simulink model "nonlin_sim_task4"  (R2023a)
settings: Solver=VariableStepAuto  StartTime=0.0  StopTime=100  RelTol=1e-3
values from neighbouring files (symbols this model uses):
  La_La_La_La_c_at_x0_numeric = double(subs(La_La_La_La_c_at_x0, param_values, param_numeric))    [nonlin_lab_task4.m]    (also in nonlin_lab_task6.m)
  Lb_La_La_La_c_at_x0_numeric = double(subs(Lb_La_La_La_c_at_x0, param_values, param_numeric))    [nonlin_lab_task4.m]    (also in nonlin_lab_task6.m)
  x_init = [0 0 0 0]'    [nonlin_lab.m]    (also in nonlin_lab_task2.m = [0 0 theta_m_eq 0]'; nonlin_lab_task4.m = [0 0 theta_m_eq 0]'; nonlin_lab_task6.m = [0 0 theta_m_eq 0]')
undefined symbols (not defined in the file or in its folder): K_lin_feedback
settings Model: Creator=M4RTI  LastModifiedBy=M4RTI

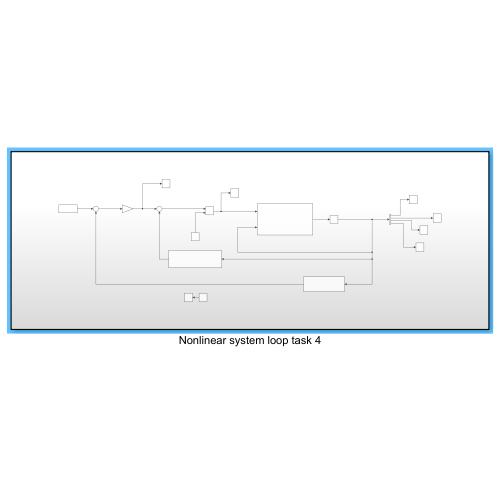
[thumbnail: Simulink's stored preview of the top-level diagram]
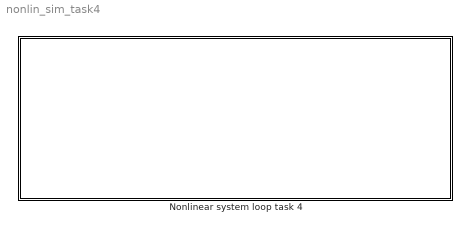
== system nonlin_sim_task4 ==
  Nonlinear system loop task 4 : Subsystem

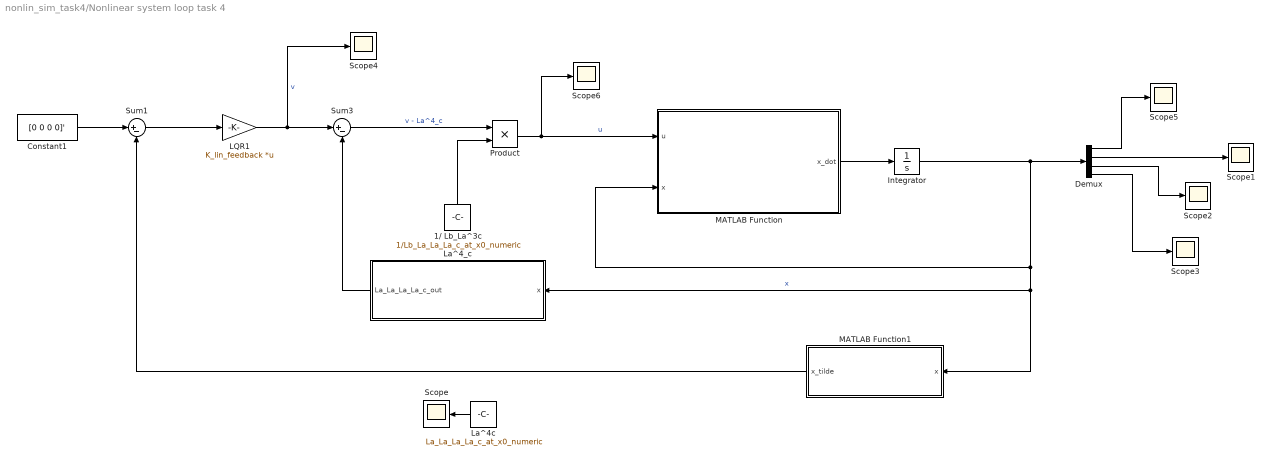
== system nonlin_sim_task4/Nonlinear system loop task 4 ==
  1/ Lb_La^3c : Constant  Value=1/Lb_La_La_La_c_at_x0_numeric
  Constant1 : Constant  Value=[0 0 0 0]'
  Demux : Demux
  Integrator : Integrator  InitialCondition=x_init
  LQR1 : Gain  Gain=K_lin_feedback  Multiplication=Matrix(K*u)
  La^4_c : MATLAB Function  TreatAsAtomicUnit=on
  La^4c : Constant  Value=La_La_La_La_c_at_x0_numeric
  MATLAB Function : MATLAB Function  TreatAsAtomicUnit=on
  MATLAB Function1 : MATLAB Function  TreatAsAtomicUnit=on
  Product : Product
  Scope{,1..6} (7 alike) : Scope
  Sum1 : Sum  Inputs=|+-
  Sum3 : Sum  Inputs=|+-
  wires:
  Demux/1 -> Scope5/1
  Demux/4 -> Scope3/1
  Integrator/1 -> Demux/1, MATLAB Function1/1(x), La^4_c/1(x), MATLAB Function/2(x)  "x"
  Demux/2 -> Scope1/1
  Demux/3 -> Scope2/1
  MATLAB Function/1(x_dot) -> Integrator/1
  Product/1 -> Scope6/1, MATLAB Function/1(u)  "u"
  LQR1/1 -> Scope4/1, Sum3/1  "v"
  Sum3/1 -> Product/1  "v - La^4_c"
  1/ Lb_La^3c/1 -> Product/2
  La^4c/1 -> Scope/1
  La^4_c/1(La_La_La_La_c_out) -> Sum3/2
  Sum1/1 -> LQR1/1
  Constant1/1 -> Sum1/1
  MATLAB Function1/1(x_tilde) -> Sum1/2

== matlab function nonlin_sim_task4/Nonlinear system loop task 4/MATLAB Function ==
  data: u input; x input; x_dot output
function x_dot = nonlin_system(u, x)
    m = 0.3;   % Mass of the load (kg)
    l = 0.3;   % Length to the center of mass of the load (m)
    g = 9.8;   % Acceleration due to gravity (m/s^2)
    J_l = 4e-4; % Moment of inertia of the load (Nms^2/rad)
    J_m = 4e-4; % Moment of inertia of the motor (Nms^2/rad)
    B_l = 0.0;  % Damping coefficient of the load (Nms/rad)
    B_m = 0.015; % Damping coefficient of the motor (Nms/rad)
    k = 0.8;    % Spring constant (Nm/rad)

    % Nonlinear dynamics
    theta_l = x(1);
    theta_l_dot = x(2);
    theta_m = x(3);
    theta_m_dot = x(4);

    x1_dot = theta_l_dot;
    x2_dot = -1/J_l * (B_l * theta_l_dot + k * (theta_l - theta_m) + m * g * l * cos(theta_l));
    x3_dot = theta_m_dot;
    x4_dot = 1/J_m * (u + k * (theta_l - theta_m) - B_m * theta_m_dot);

    % Output: the derivatives of the state variables
    x_dot = [x1_dot; x2_dot; x3_dot; x4_dot];
end

== matlab function nonlin_sim_task4/Nonlinear system loop task 4/La^4_c ==
  data: x input; La_La_La_La_c_out output
function La_La_La_La_c_out = computeLaLaLaLaC(x)
    m = 0.3;   % Mass of the load (kg)
    l = 0.3;   % Length to the center of mass of the load (m)
    g = 9.8;   % Acceleration due to gravity (m/s^2)
    J_l = 4e-4; % Moment of inertia of the load (Nms^2/rad)
    J_m = 4e-4; % Moment of inertia of the motor (Nms^2/rad)
    B_l = 0.0;  % Damping coefficient of the load (Nms/rad)
    B_m = 0.015; % Damping coefficient of the motor (Nms/rad)
    k = 0.8;    % Spring constant (Nm/rad)

    % Extract state variables from x
    theta_l = x(1);
    theta_l_dot = x(2);
    theta_m = x(3);
    theta_m_dot = x(4);

    % Compute La_La_La_La_c
    La_La_La_La_c_out = ((k*(theta_l - theta_m))/J_l + (B_l*theta_l_dot)/J_l + (g*l*m*cos(theta_l))/J_l)*(B_l^2/J_l^2 - k/J_l + (g*l*m*sin(theta_l))/J_l) - theta_l_dot*((B_l*(k/J_l - (g*l*m*sin(theta_l))/J_l))/J_l + (g*l*m*theta_l_dot*cos(theta_l))/J_l) - (k*((k*(theta_l - theta_m))/J_m - (B_m*theta_m_dot)/J_m))/J_l + (B_l*k*theta_m_dot)/J_l^2;
end

== matlab function nonlin_sim_task4/Nonlinear system loop task 4/MATLAB Function1 ==
  data: x input; x_tilde output
function x_tilde = transform_to_x_tilde(x)
    % Transformation from x to x_tilde = [y; y_dot; y_dot_dot; y_dot_dot_dot]
    m = 0.3;   % Mass of the load (kg)
    l = 0.3;   % Length to the center of mass of the load (m)
    g = 9.8;   % Acceleration due to gravity (m/s^2)
    J_l = 4e-4; % Moment of inertia of the load (Nms^2/rad)
    J_m = 4e-4; % Moment of inertia of the motor (Nms^2/rad)
    B_l = 0.0;  % Damping coefficient of the load (Nms/rad)
    B_m = 0.015; % Damping coefficient of the motor (Nms/rad)
    k = 0.8;    % Spring constant (Nm/rad)
    
    x_tilde_1 = pi/4 - x(1);
    x_tilde_2 = -x(2);
    x_tilde_3 = (k*(x(1) - x(3)))/J_l + (B_l*x(2))/J_l + (g*l*m*cos(x(1)))/J_l;
    x_tilde_4 = x(2)*(k/J_l - (g*l*m*sin(x(1)))/J_l) - (B_l*((k*(x(1) - x(3)))/J_l + (B_l*x(2))/J_l + (g*l*m*cos(x(1)))/J_l))/J_l - (k*x(4))/J_l;
    
    x_tilde = [x_tilde_1; x_tilde_2; x_tilde_3; x_tilde_4];
end
